simulink model "testOpenLoop"  (R2021a)
settings: Solver=VariableStepAuto  StartTime=0.0  StopTime=200  RelTol=1e-3
libraries: sharedtransform x1
settings Model: DataDictionary=databus.sldd  Creator=Laura  LastModifiedBy=Laura

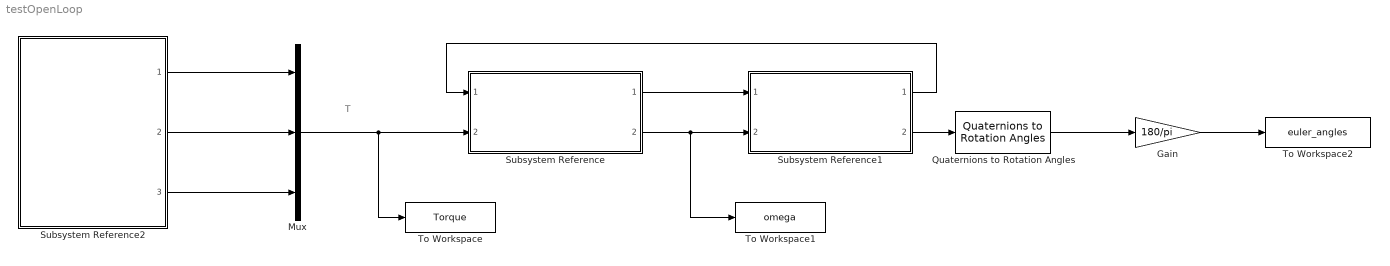
== system testOpenLoop ==
  note: T
  Gain : Gain  Gain=180/pi
  Mux : Mux  Inputs=3
  Quaternions to Rotation Angles : sharedtransform/Quaternions to Rotation Angles  rotationOrder=ZYX  aMode=aMode
      settings: SourceProductBaseCode=AE,PW,DR,MT,UV,VE
  Subsystem Reference : Subsystem  ReferencedSubsystem=Dynamics
  Subsystem Reference1 : Subsystem  ReferencedSubsystem=Kinematics
  Subsystem Reference2 : Subsystem  ReferencedSubsystem=ThrustSignals
  To Workspace : ToWorkspace  VariableName=Torque  SaveFormat=Timeseries  SampleTime=-1
  To Workspace1 : ToWorkspace  VariableName=omega  SaveFormat=Timeseries  SampleTime=-1
  To Workspace2 : ToWorkspace  VariableName=euler_angles  SaveFormat=Timeseries  SampleTime=-1
  wires:
  Subsystem Reference1/1 -> Subsystem Reference/1
  Subsystem Reference1/2 -> Quaternions to Rotation Angles/1
  Subsystem Reference/2 -> To Workspace1/1, Subsystem Reference1/2
  Subsystem Reference/1 -> Subsystem Reference1/1
  Mux/1 -> To Workspace/1, Subsystem Reference/2
  Quaternions to Rotation Angles/1 -> Gain/1
  Subsystem Reference2/2 -> Mux/2
  Subsystem Reference2/1 -> Mux/1
  Subsystem Reference2/3 -> Mux/3
  Gain/1 -> To Workspace2/1
